simulink model "lqr"  (R2022b)
settings: Solver=FixedStepAuto  StartTime=0.0  StopTime=100  FixedStep=0.01  RelTol=1e-3
undefined symbols (not defined in the file or in its folder): K_LQR
settings Model: Creator=mehti  LastModifiedBy=MMM
settings SolverCC: AlgebraicLoopSolver=TrustRegion
settings DebuggingCC: UnconnectedInputMsg=warning  UnconnectedOutputMsg=warning  UnconnectedLineMsg=warning  SFMachineParentedDataDiag=warning
settings ModelReferenceCC: EnableRefExpFcnMdlSchedulingChecks=on
settings RTWCC: DLArmComputeVersion=19.05

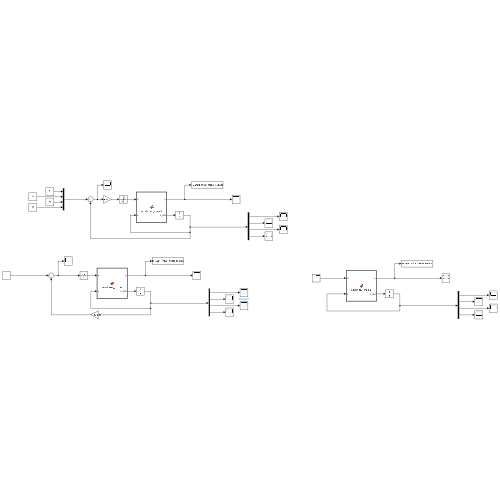
[thumbnail: Simulink's stored preview of the top-level diagram]
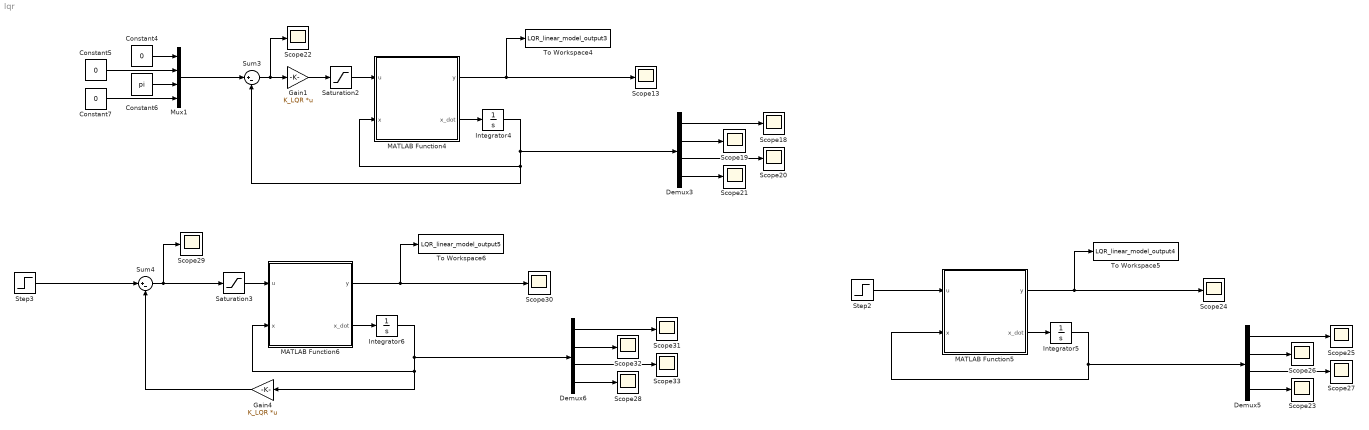
== system lqr ==
  Constant4 : Constant  Value=0
  Constant5 : Constant  Value=0
  Constant6 : Constant  Value=pi
  Constant7 : Constant  Value=0
  Demux3 : Demux
  Demux5 : Demux
  Demux6 : Demux
  Gain1 : Gain  Gain=K_LQR  Multiplication=Matrix(K*u)
  Gain4 : Gain  Gain=K_LQR  Multiplication=Matrix(K*u)
  Integrator4 : Integrator  InitialCondition=[0, 0, pi + pi/8 ,0]
  Integrator5 : Integrator  InitialCondition=[0, 0, pi + pi/8 ,0]
  Integrator6 : Integrator  InitialCondition=[0, 0, pi + pi/8 ,0]
  MATLAB Function4 : MATLAB Function  TreatAsAtomicUnit=on
  MATLAB Function5 : MATLAB Function  TreatAsAtomicUnit=on
  MATLAB Function6 : MATLAB Function  TreatAsAtomicUnit=on
  Mux1 : Mux
  Saturation2 : Saturate  UpperLimit=10  LowerLimit=-10
  Saturation3 : Saturate  UpperLimit=10  LowerLimit=-10
  Scope{13,18..33} (17 alike) : Scope
  Step2 : Step  Time=0.5  After=0  SampleTime=0
  Step3 : Step  Time=0.5  After=0.2  SampleTime=0
  Sum3 : Sum  Inputs=|+-
  Sum4 : Sum  Inputs=|+-
  To Workspace4 : ToWorkspace  VariableName=LQR_linear_model_output3  SaveFormat=Timeseries  SampleTime=-1
  To Workspace5 : ToWorkspace  VariableName=LQR_linear_model_output4  SaveFormat=Timeseries  SampleTime=-1
  To Workspace6 : ToWorkspace  VariableName=LQR_linear_model_output5  SaveFormat=Timeseries  SampleTime=-1
  wires:
  Saturation2/1 -> MATLAB Function4/1(u)
  Constant7/1 -> Mux1/4
  Constant5/1 -> Mux1/2
  Constant6/1 -> Mux1/3
  Constant4/1 -> Mux1/1
  Demux3/1 -> Scope18/1
  Demux3/2 -> Scope19/1
  Demux3/3 -> Scope20/1
  Demux3/4 -> Scope21/1
  Gain1/1 -> Saturation2/1
  Integrator4/1 -> MATLAB Function4/2(x), Sum3/2, Demux3/1
  Sum3/1 -> Gain1/1, Scope22/1
  MATLAB Function4/2(x_dot) -> Integrator4/1
  MATLAB Function4/1(y) -> To Workspace4/1, Scope13/1
  Mux1/1 -> Sum3/1
  Step2/1 -> MATLAB Function5/1(u)
  Demux5/1 -> Scope25/1
  Demux5/2 -> Scope26/1
  Demux5/3 -> Scope27/1
  MATLAB Function5/2(x_dot) -> Integrator5/1
  Integrator5/1 -> Demux5/1, MATLAB Function5/2(x)
  Demux5/4 -> Scope23/1
  MATLAB Function5/1(y) -> Scope24/1, To Workspace5/1
  Step3/1 -> Sum4/1
  Gain4/1 -> Sum4/2
  MATLAB Function6/1(y) -> To Workspace6/1, Scope30/1
  Demux6/4 -> Scope28/1
  Integrator6/1 -> MATLAB Function6/2(x), Gain4/1, Demux6/1
  MATLAB Function6/2(x_dot) -> Integrator6/1
  Demux6/3 -> Scope33/1
  Demux6/2 -> Scope32/1
  Saturation3/1 -> MATLAB Function6/1(u)
  Demux6/1 -> Scope31/1
  Sum4/1 -> Scope29/1, Saturation3/1

== matlab function lqr/MATLAB Function4 ==
  data: u input; y output; x input; x_dot output
function [y, x_dot] = nonlinear_model(u, x)

% The state variables
x1 = x(1); x2 = x(2);
x3 = x(3); x4 = x(4);

% Parameters
m = 1;       % Pendulum mass [kg]
M = 5;       % Cart mass [kg]
L = 2;       % Pendulum length [m]
g = 9.8065;  % Gravitational acceleration [m/s^2]
d = 1;       % Coefficient

D = m * L^2 * (M + m * (1 - cos(x3)^2));

% Nonlinear equations 
x_dot = [x2;
         (1/D) * (-m^2*L^2*g*cos(x3)*sin(x3) + m*L^2*(m*L*x4^2*sin(x3)...
         - d*x2) + m*L^2*u);
         x4;
        (1/D) * ((m+M)*m*g*L*sin(x3) - m*L*cos(x3)*(m*L*x4^2*sin(x3)...
        - d*x2) - m*L*cos(x3)*u) 
         ];

y = [x1;
     x3];

end

== matlab function lqr/MATLAB Function5 ==
  data: u input; y output; x input; x_dot output
function [y, x_dot] = nonlinear_model(u, x)

% The state variables
x1 = x(1); x2 = x(2);
x3 = x(3); x4 = x(4);

% Parameters
m = 1;       % Pendulum mass [kg]
M = 5;       % Cart mass [kg]
L = 2;       % Pendulum length [m]
g = 9.8065;  % Gravitational acceleration [m/s^2]
d = 1;       % Coefficient

D = m * L^2 * (M + m * (1 - cos(x3)^2));

% Nonlinear equations 
x_dot = [x2;
         (1/D) * (-m^2*L^2*g*cos(x3)*sin(x3) + m*L^2*(m*L*x4^2*sin(x3)...
         - d*x2) + m*L^2*u);
         x4;
        (1/D) * ((m+M)*m*g*L*sin(x3) - m*L*cos(x3)*(m*L*x4^2*sin(x3)...
        - d*x2) - m*L*cos(x3)*u) 
         ];

y = [x1;
     x3];

end

== matlab function lqr/MATLAB Function6 ==
  data: u input; y output; x input; x_dot output
function [y, x_dot] = nonlinear_model(u, x)

% The state variables
x1 = x(1); x2 = x(2);
x3 = x(3); x4 = x(4);

% Parameters
m = 1;       % Pendulum mass [kg]
M = 5;       % Cart mass [kg]
L = 2;       % Pendulum length [m]
g = 9.8065;  % Gravitational acceleration [m/s^2]
d = 1;       % Coefficient

D = m * L^2 * (M + m * (1 - cos(x3)^2));

% Nonlinear equations 
x_dot = [x2;
         (1/D) * (-m^2*L^2*g*cos(x3)*sin(x3) + m*L^2*(m*L*x4^2*sin(x3)...
         - d*x2) + m*L^2*u);
         x4;
        (1/D) * ((m+M)*m*g*L*sin(x3) - m*L*cos(x3)*(m*L*x4^2*sin(x3)...
        - d*x2) - m*L*cos(x3)*u) 
         ];

y = [x1;
     x3];

end
